simulink model "proto1"  (R2013b)
settings: Solver=ode45  StartTime=0.0  StopTime=20  RelTol=1e-3
libraries: xbsIndex_r4 x145, xps_library x1
settings Model: Creator=root  LastModifiedBy=root

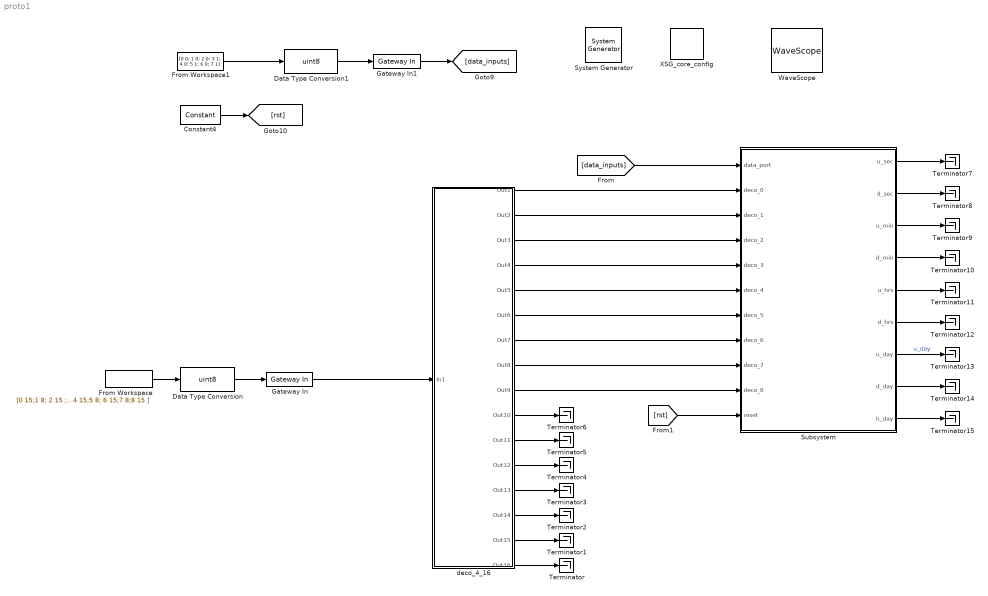
== system proto1 ==
  " System Generator" : xbsIndex_r4/ System Generator  Tag=genX  xilinxfamily=Kintex7  part=xc7k325t  speed=-3  package=fbg676  synthesis_tool=XST  clock_wrapper=Clock Enables  directory=./netlist  proj_type=Project Navigator  Synth_file=XST Defaults  Impl_file=ISE Defaults  testbench=off  simulink_period=1  sysclk_period=10  dcm_input_clock_period=10  incr_netlist=off  trim_vbits=Everywhere in SubSystem  dbl_ovrd=According to Block Masks  core_generation=According to Block Masks  run_coregen=off  deprecated_control=off  eval_field=0  block_type=sysgen
  Constant4 : xbsIndex_r4/Constant  const=0  gui_display_data_type=Boolean  arith_type=Boolean  n_bits=16  bin_pt=14  preci_type=Single  exp_width=8  frac_width=24  explicit_period=on  period=1  equ=P=C  opselect=C  inp2=PCIN>>17  opr=+  inp1=P  carry=CIN  dbl_ovrd=off  block_type=constant
  Data Type Conversion : DataTypeConversion  OutDataTypeStr=uint8
  Data Type Conversion1 : DataTypeConversion  OutDataTypeStr=uint8
  From Workspace : FromWorkspace  VariableName=[0 15;1 8; 2 15 ;3 8; 4 15;5 8; 6 15;7 8;8 15 ]  OutDataTypeStr=double  SampleTime=0  OutputAfterFinalValue=Holding final value
  From Workspace1 : FromWorkspace  VariableName=[0 0; 1 0; 2 0; 3 1; 4 0; 5 1; 6 0; 7 1]  OutDataTypeStr=double  SampleTime=0  OutputAfterFinalValue=Holding final value
  Gateway In : xbsIndex_r4/Gateway In  gui_display_data_type=Fixed-point  arith_type=Unsigned  n_bits=8  bin_pt=0  preci_type=Single  exp_width=8  frac_width=24  quantization="Round  (unbiased: +/- Inf)"  overflow=Saturate  period=1  dbl_ovrd=off  timing_constraint=None  locs_specified=off  LOCs={}  UseAsADC=off  ADCChannel='1'  inherit_from_input=off  hdl_port=on  block_type=gatewayin
  Gateway In1 : xbsIndex_r4/Gateway In  gui_display_data_type=Fixed-point  arith_type=Unsigned  n_bits=8  bin_pt=0  preci_type=Single  exp_width=8  frac_width=24  quantization="Round  (unbiased: +/- Inf)"  overflow=Saturate  period=1  dbl_ovrd=off  timing_constraint=None  locs_specified=off  LOCs={}  UseAsADC=off  ADCChannel='1'  inherit_from_input=off  hdl_port=on  block_type=gatewayin
  Subsystem : Subsystem
  Terminator{,1..15} (16 alike) : Terminator
  WaveScope : xbsIndex_r4/WaveScope  block_type=wavescope
  XSG_core_config : xps_library/XSG_core_config  Tag=xps:xsg  hw_sys=ROACH2:sx475t  clk_src=sys_clk  ROACH_clk_src=sys_clk  ROACH2_clk_src=sys_clk  MKDIG_clk_src=sys_clk  clk_rate=100  sample_period=1  synthesis_tool=XST
  deco_4_16 : Subsystem
  wires:
  From Workspace/1 -> Data Type Conversion/1
  Data Type Conversion/1 -> Gateway In/1
  Gateway In/1 -> deco_4_16/1(In1)
  deco_4_16/16(Out16) -> Terminator/1
  deco_4_16/15(Out15) -> Terminator1/1
  deco_4_16/14(Out14) -> Terminator2/1
  deco_4_16/13(Out13) -> Terminator3/1
  deco_4_16/12(Out12) -> Terminator4/1
  deco_4_16/11(Out11) -> Terminator5/1
  deco_4_16/10(Out10) -> Terminator6/1
  deco_4_16/1(Out1) -> Subsystem/2(deco_0)
  deco_4_16/2(Out2) -> Subsystem/3(deco_1)
  deco_4_16/3(Out3) -> Subsystem/4(deco_2)
  deco_4_16/4(Out4) -> Subsystem/5(deco_3)
  deco_4_16/5(Out5) -> Subsystem/6(deco_4)
  deco_4_16/6(Out6) -> Subsystem/7(deco_5)
  deco_4_16/7(Out7) -> Subsystem/8(deco_6)
  deco_4_16/8(Out8) -> Subsystem/9(deco_7)
  deco_4_16/9(Out9) -> Subsystem/10(deco_8)
  From Workspace1/1 -> Data Type Conversion1/1
  Data Type Conversion1/1 -> Gateway In1/1
  Gateway In1/1 -> [data_inputs]
  Constant4/1 -> [rst]
  [data_inputs] -> Subsystem/1(data_port)
  [rst] -> Subsystem/11(reset)
  Subsystem/1(u_sec) -> Terminator7/1
  Subsystem/2(d_sec) -> Terminator8/1
  Subsystem/3(u_min) -> Terminator9/1
  Subsystem/4(d_min) -> Terminator10/1
  Subsystem/5(u_hrs) -> Terminator11/1
  Subsystem/6(d_hrs) -> Terminator12/1
  Subsystem/7(u_day) -> Terminator13/1  "u_day"
  Subsystem/8(d_day) -> Terminator14/1
  Subsystem/9(h_day) -> Terminator15/1

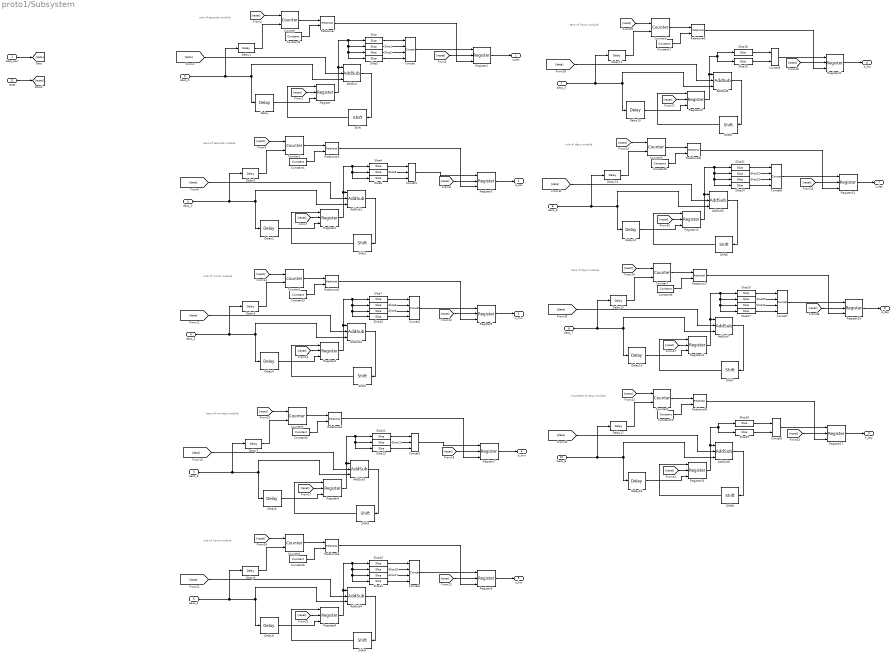
== system proto1/Subsystem ==
  note: unit of seconds module
  note: tens of seconds module
  note: unit of minits module
  note: tens of minutes module
  note: unit of hours module
  note: tens of hours module
  note: unit of days module
  note: tens of days module
  note: houdreds of days module
  data_port : Inport
  deco_0 : Inport  Port=2
  deco_1 : Inport  Port=3
  deco_2 : Inport  Port=4
  deco_3 : Inport  Port=5
  deco_4 : Inport  Port=6
  deco_5 : Inport  Port=7
  deco_6 : Inport  Port=8
  deco_7 : Inport  Port=9
  deco_8 : Inport  Port=10
  reset : Inport  Port=11
  AddSub{,2,4,6..7} (5 alike) : xbsIndex_r4/AddSub  mode=Addition  use_carryin=off  use_carryout=off  en=on  latency=1  precision=User Defined  arith_type=Unsigned  n_bits=5  bin_pt=0  quantization=Truncate  overflow=Wrap  dbl_ovrd=off  use_behavioral_HDL=off  hw_selection=Fabric  pipelined=off  block_type=addsub
  AddSub1 : xbsIndex_r4/AddSub  mode=Addition  use_carryin=off  use_carryout=off  en=on  latency=1  precision=User Defined  arith_type=Unsigned  n_bits=4  bin_pt=0  quantization=Truncate  overflow=Wrap  dbl_ovrd=off  use_behavioral_HDL=off  hw_selection=Fabric  pipelined=off  block_type=addsub
  AddSub3 : xbsIndex_r4/AddSub  mode=Addition  use_carryin=off  use_carryout=off  en=on  latency=1  precision=User Defined  arith_type=Unsigned  n_bits=4  bin_pt=0  quantization=Truncate  overflow=Wrap  dbl_ovrd=off  use_behavioral_HDL=off  hw_selection=Fabric  pipelined=off  block_type=addsub
  AddSub5 : xbsIndex_r4/AddSub  mode=Addition  use_carryin=off  use_carryout=off  en=on  latency=1  precision=User Defined  arith_type=Unsigned  n_bits=3  bin_pt=0  quantization=Truncate  overflow=Wrap  dbl_ovrd=off  use_behavioral_HDL=off  hw_selection=Fabric  pipelined=off  block_type=addsub
  AddSub8 : xbsIndex_r4/AddSub  mode=Addition  use_carryin=off  use_carryout=off  en=on  latency=1  precision=User Defined  arith_type=Unsigned  n_bits=3  bin_pt=0  quantization=Truncate  overflow=Wrap  dbl_ovrd=off  use_behavioral_HDL=off  hw_selection=Fabric  pipelined=off  block_type=addsub
  Concat{,2,4,6..7} (5 alike) : xbsIndex_r4/Concat  num_inputs=4  dbl_ovrd=off  block_type=concat
  Concat1 : xbsIndex_r4/Concat  num_inputs=3  dbl_ovrd=off  block_type=concat
  Concat3 : xbsIndex_r4/Concat  num_inputs=3  dbl_ovrd=off  block_type=concat
  Concat5 : xbsIndex_r4/Concat  num_inputs=2  dbl_ovrd=off  block_type=concat
  Concat8 : xbsIndex_r4/Concat  num_inputs=2  dbl_ovrd=off  block_type=concat
  Constant1 : xbsIndex_r4/Constant  const=3  gui_display_data_type=Fixed-point  arith_type=Unsigned  n_bits=4  bin_pt=0  preci_type=Single  exp_width=8  frac_width=24  explicit_period=on  period=1  equ=P=C  opselect=C  inp2=PCIN>>17  opr=+  inp1=P  carry=CIN  dbl_ovrd=off  block_type=constant
  Constant10 : xbsIndex_r4/Constant  const=2  gui_display_data_type=Fixed-point  arith_type=Unsigned  n_bits=3  bin_pt=0  preci_type=Single  exp_width=8  frac_width=24  explicit_period=on  period=1  equ=P=C  opselect=C  inp2=PCIN>>17  opr=+  inp1=P  carry=CIN  dbl_ovrd=off  block_type=constant
  Constant{2..3,6,8..9} (5 alike) : xbsIndex_r4/Constant  const=4  gui_display_data_type=Fixed-point  arith_type=Unsigned  n_bits=4  bin_pt=0  preci_type=Single  exp_width=8  frac_width=24  explicit_period=on  period=1  equ=P=C  opselect=C  inp2=PCIN>>17  opr=+  inp1=P  carry=CIN  dbl_ovrd=off  block_type=constant
  Constant5 : xbsIndex_r4/Constant  const=3  gui_display_data_type=Fixed-point  arith_type=Unsigned  n_bits=4  bin_pt=0  preci_type=Single  exp_width=8  frac_width=24  explicit_period=on  period=1  equ=P=C  opselect=C  inp2=PCIN>>17  opr=+  inp1=P  carry=CIN  dbl_ovrd=off  block_type=constant
  Constant7 : xbsIndex_r4/Constant  const=2  gui_display_data_type=Fixed-point  arith_type=Unsigned  n_bits=3  bin_pt=0  preci_type=Single  exp_width=8  frac_width=24  explicit_period=on  period=1  equ=P=C  opselect=C  inp2=PCIN>>17  opr=+  inp1=P  carry=CIN  dbl_ovrd=off  block_type=constant
  Counter{,1..8} (9 alike) : xbsIndex_r4/Counter  cnt_type=Free Running  cnt_to=Inf  operation=Up  start_count=0  cnt_by_val=1  arith_type=Unsigned  n_bits=4  bin_pt=0  load_pin=off  rst=on  en=on  explicit_period=on  period=1  dbl_ovrd=off  use_behavioral_HDL=off  implementation=Fabric  block_type=counter
  Delay{,1..17} (18 alike) : xbsIndex_r4/Delay  rst=off  infoeditControl=Selection of Reset will increase slice count due to use of real FFs and instead of SRLs  en=off  latency=1  dbl_ovrd=off  reg_retiming=off  block_type=delay
  Register{,1..17} (18 alike) : xbsIndex_r4/Register  init=0  rst=on  en=on  dbl_ovrd=off  block_type=register
  Relational{,1..8} (9 alike) : xbsIndex_r4/Relational  mode=a=b  en=off  latency=0  dbl_ovrd=off  block_type=relational
  Shift{,1..8} (9 alike) : xbsIndex_r4/Shift  shift_dir=Left  shift_bits=1  en=off  latency=0  precision=Full  arith_type="Signed  (2's comp)"  n_bits=16  bin_pt=14  quantization=Truncate  overflow=Wrap  dbl_ovrd=off  block_type=shift
  Slice{,4,7,11,15,18,20..21,28} (9 alike) : xbsIndex_r4/Slice  nbits=1  boolean_output=off  mode=Lower Bit Location + Width  bit1=0  base1=MSB of Input  bit0=1  base0=LSB of Input  dbl_ovrd=off  block_type=slice
  Slice{1,5,8,12,16,19,22,25,29} (9 alike) : xbsIndex_r4/Slice  nbits=1  boolean_output=off  mode=Lower Bit Location + Width  bit1=0  base1=MSB of Input  bit0=2  base0=LSB of Input  dbl_ovrd=off  block_type=slice
  Slice{3,10,14,24,27} (5 alike) : xbsIndex_r4/Slice  nbits=1  boolean_output=off  mode=Lower Bit Location + Width  bit1=0  base1=MSB of Input  bit0=4  base0=LSB of Input  dbl_ovrd=off  block_type=slice
  Slice{2,6,9,13,17,23,26} (7 alike) : xbsIndex_r4/Slice  nbits=1  boolean_output=off  mode=Lower Bit Location + Width  bit1=0  base1=MSB of Input  bit0=3  base0=LSB of Input  dbl_ovrd=off  block_type=slice
  u_sec : Outport
  d_sec : Outport  Port=2
  u_min : Outport  Port=3
  d_min : Outport  Port=4
  u_hrs : Outport  Port=5
  d_hrs : Outport  Port=6
  u_day : Outport  Port=7
  d_day : Outport  Port=8
  h_day : Outport  Port=9
  wires:
  Constant7/1 -> Relational5/2
  Shift7/1 -> Register14/1
  Delay14/1 -> Register14/3
  [reset] -> Register10/2
  deco_5/1 -> Delay11/1, Delay10/1, AddSub5/3
  Register12/1 -> Slice24/1, Slice23/1, Slice22/1, Slice21/1, AddSub6/1
  Shift5/1 -> Register10/1
  Relational5/1 -> Register11/3
  [reset] -> Counter5/1
  Register15/1 -> d_day/1
  Delay15/1 -> Counter7/2
  [data] -> AddSub1/2
  Register13/1 -> u_day/1
  Delay13/1 -> Counter6/2
  Slice24/1 -> Concat6/4
  Register11/1 -> d_hrs/1
  [data] -> AddSub5/2
  AddSub5/1 -> Shift5/1
  Slice21/1 -> Concat6/1
  Slice23/1 -> Concat6/3
  Slice22/1 -> Concat6/2
  Register5/1 -> u_min/1
  Shift2/1 -> Register4/1
  [reset] -> Register3/2
  Slice7/1 -> Concat2/1
  Slice8/1 -> Concat2/2
  Delay6/1 -> Register6/3
  Slice12/1 -> Concat3/2
  [data] -> AddSub7/2
  [reset] -> Register11/2
  Register3/1 -> d_sec/1
  Counter7/1 -> Relational7/1
  Delay/1 -> Register/3
  Slice/1 -> Concat/1
  Slice1/1 -> Concat/2
  Slice2/1 -> Concat/3
  Concat/1 -> Register1/1
  [reset] -> Counter/1
  Counter/1 -> Relational/1
  Constant2/1 -> Relational/2
  Relational/1 -> Register1/3
  [reset] -> Register1/2
  Register1/1 -> u_sec/1
  Delay1/1 -> Counter/2
  Slice6/1 -> Concat1/3
  [reset] -> Counter2/1
  Slice27/1 -> Concat7/4
  Slice20/1 -> Concat7/1
  Slice25/1 -> Concat7/2
  Slice26/1 -> Concat7/3
  Relational8/1 -> Register17/3
  [reset] -> Register17/2
  Register17/1 -> h_day/1
  Delay17/1 -> Counter8/2
  Register8/1 -> Slice14/1, Slice17/1, Slice16/1, Slice15/1, AddSub4/1
  [reset] -> Register12/2
  Shift6/1 -> Register12/1
  Delay12/1 -> Register12/3
  Delay10/1 -> Register10/3
  Slice29/1 -> Concat8/2
  Concat8/1 -> Register17/1
  [reset] -> Counter8/1
  Counter8/1 -> Relational8/1
  Constant10/1 -> Relational8/2
  AddSub8/1 -> Shift8/1
  Shift8/1 -> Register16/1
  Delay16/1 -> Register16/3
  Slice28/1 -> Concat8/1
  [reset] -> Register15/2
  deco_8/1 -> Delay17/1, AddSub8/3, Delay16/1
  [data] -> AddSub8/2
  [reset] -> Register16/2
  Register14/1 -> Slice27/1, Slice26/1, Slice25/1, Slice20/1, AddSub7/1
  Constant9/1 -> Relational7/2
  Relational7/1 -> Register15/3
  AddSub7/1 -> Shift7/1
  [reset] -> Register14/2
  Register16/1 -> Slice29/1, Slice28/1, AddSub8/1
  Register2/1 -> Slice6/1, Slice5/1, Slice4/1, AddSub1/1
  Constant5/1 -> Relational3/2
  [reset] -> Register7/2
  Slice19/1 -> Concat5/2
  [reset] -> Register2/2
  Constant1/1 -> Relational1/2
  AddSub2/1 -> Shift2/1
  [reset] -> Register4/2
  Concat7/1 -> Register15/1
  [reset] -> Counter7/1
  deco_2/1 -> Delay5/1, Delay4/1, AddSub2/3
  [data] -> AddSub3/2
  Delay4/1 -> Register4/3
  Slice9/1 -> Concat2/3
  Counter1/1 -> Relational1/1
  Counter5/1 -> Relational5/1
  Concat1/1 -> Register3/1
  Slice3/1 -> Concat/4
  Shift3/1 -> Register6/1
  AddSub3/1 -> Shift3/1
  Register10/1 -> Slice19/1, Slice18/1, AddSub5/1
  Relational2/1 -> Register5/3
  [reset] -> Register5/2
  AddSub1/1 -> Shift1/1
  Delay7/1 -> Counter3/2
  [data] -> AddSub6/2
  AddSub6/1 -> Shift6/1
  Relational3/1 -> Register7/3
  Register7/1 -> d_min/1
  deco_3/1 -> Delay7/1, Delay6/1, AddSub3/3
  Counter3/1 -> Relational3/1
  [reset] -> Counter3/1
  Slice10/1 -> Concat2/4
  Delay5/1 -> Counter2/2
  [data] -> AddSub2/2
  Relational1/1 -> Register3/3
  Counter2/1 -> Relational2/1
  Constant3/1 -> Relational2/2
  [reset] -> Register9/2
  Register9/1 -> u_hrs/1
  Delay9/1 -> Counter4/2
  Slice14/1 -> Concat4/4
  Register/1 -> Slice3/1, Slice2/1, Slice1/1, Slice/1, AddSub/1
  Register6/1 -> Slice13/1, Slice12/1, Slice11/1, AddSub3/1
  Concat2/1 -> Register5/1
  Delay3/1 -> Counter1/2
  Register4/1 -> Slice10/1, Slice9/1, Slice8/1, Slice7/1, AddSub2/1
  [reset] -> Counter4/1
  deco_6/1 -> Delay13/1, AddSub6/3, Delay12/1
  [data] -> AddSub4/2
  AddSub4/1 -> Shift4/1
  [reset] -> Register8/2
  deco_4/1 -> Delay9/1, Delay8/1, AddSub4/3
  Concat5/1 -> Register11/1
  Constant8/1 -> Relational6/2
  [reset] -> Register13/2
  Relational6/1 -> Register13/3
  Slice17/1 -> Concat4/3
  Constant6/1 -> Relational4/2
  Counter4/1 -> Relational4/1
  Relational4/1 -> Register9/3
  Delay11/1 -> Counter5/2
  Concat6/1 -> Register13/1
  Counter6/1 -> Relational6/1
  [reset] -> Counter6/1
  Slice18/1 -> Concat5/1
  deco_7/1 -> Delay15/1, Delay14/1, AddSub7/3
  Shift4/1 -> Register8/1
  Delay8/1 -> Register8/3
  Slice15/1 -> Concat4/1
  Concat4/1 -> Register9/1
  Slice16/1 -> Concat4/2
  Slice13/1 -> Concat3/3
  Concat3/1 -> Register7/1
  deco_1/1 -> Delay3/1, Delay2/1, AddSub1/3
  Delay2/1 -> Register2/3
  deco_0/1 -> Delay1/1, Delay/1, AddSub/3
  [data] -> AddSub/2
  AddSub/1 -> Shift/1
  [reset] -> Register/2
  Shift/1 -> Register/1
  Slice5/1 -> Concat1/2
  Shift1/1 -> Register2/1
  Slice4/1 -> Concat1/1
  [reset] -> Register6/2
  Slice11/1 -> Concat3/1
  [reset] -> Counter1/1
  data_port/1 -> [data]
  reset/1 -> [reset]

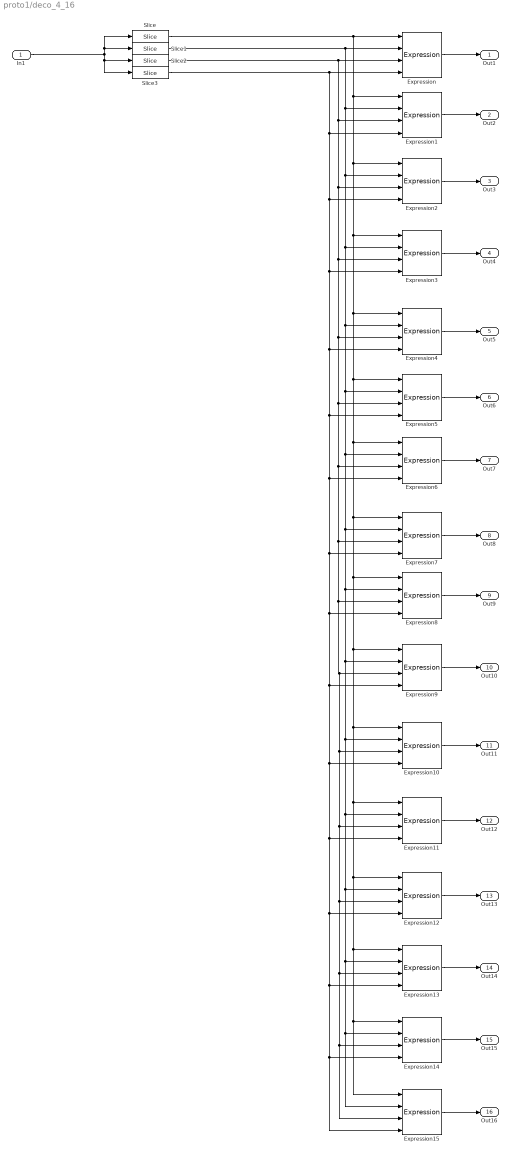
== system proto1/deco_4_16 ==
  In1 : Inport
  Expression : xbsIndex_r4/Expression  expression=~a & ~b & ~c & ~d  align_bp=on  en=off  latency=0  precision=Full  arith_type=Unsigned  n_bits=16  bin_pt=0  dbl_ovrd=off  block_type=expr
  Expression1 : xbsIndex_r4/Expression  expression=~a & ~b & ~c & d  align_bp=on  en=off  latency=0  precision=Full  arith_type=Unsigned  n_bits=16  bin_pt=0  dbl_ovrd=off  block_type=expr
  Expression10 : xbsIndex_r4/Expression  expression=a & ~b & c & ~d  align_bp=on  en=off  latency=0  precision=Full  arith_type=Unsigned  n_bits=16  bin_pt=0  dbl_ovrd=off  block_type=expr
  Expression11 : xbsIndex_r4/Expression  expression=a & ~b & c & d  align_bp=on  en=off  latency=0  precision=Full  arith_type=Unsigned  n_bits=16  bin_pt=0  dbl_ovrd=off  block_type=expr
  Expression12 : xbsIndex_r4/Expression  expression=a & b & ~c & ~d  align_bp=off  en=off  latency=0  precision=Full  arith_type=Unsigned  n_bits=16  bin_pt=0  dbl_ovrd=off  block_type=expr
  Expression13 : xbsIndex_r4/Expression  expression=a & b & ~c & d  align_bp=off  en=off  latency=0  precision=Full  arith_type=Unsigned  n_bits=16  bin_pt=0  dbl_ovrd=off  block_type=expr
  Expression14 : xbsIndex_r4/Expression  expression=a & b & c & ~d  align_bp=off  en=off  latency=0  precision=Full  arith_type=Unsigned  n_bits=16  bin_pt=0  dbl_ovrd=off  block_type=expr
  Expression15 : xbsIndex_r4/Expression  expression=a & b & c & d  align_bp=off  en=off  latency=0  precision=Full  arith_type=Unsigned  n_bits=16  bin_pt=0  dbl_ovrd=off  block_type=expr
  Expression2 : xbsIndex_r4/Expression  expression=~a & ~b & c & ~d  align_bp=on  en=off  latency=0  precision=Full  arith_type=Unsigned  n_bits=16  bin_pt=0  dbl_ovrd=off  block_type=expr
  Expression3 : xbsIndex_r4/Expression  expression=~a & ~b & c & d  align_bp=on  en=off  latency=0  precision=Full  arith_type=Unsigned  n_bits=16  bin_pt=0  dbl_ovrd=off  block_type=expr
  Expression4 : xbsIndex_r4/Expression  expression=~a & b & ~c & ~d  align_bp=on  en=off  latency=0  precision=Full  arith_type=Unsigned  n_bits=16  bin_pt=0  dbl_ovrd=off  block_type=expr
  Expression5 : xbsIndex_r4/Expression  expression=~a & b & ~c & d  align_bp=on  en=off  latency=0  precision=Full  arith_type=Unsigned  n_bits=16  bin_pt=0  dbl_ovrd=off  block_type=expr
  Expression6 : xbsIndex_r4/Expression  expression=~a & b & c & ~d  align_bp=on  en=off  latency=0  precision=Full  arith_type=Unsigned  n_bits=16  bin_pt=0  dbl_ovrd=off  block_type=expr
  Expression7 : xbsIndex_r4/Expression  expression=~a & b & c & d  align_bp=on  en=off  latency=0  precision=Full  arith_type=Unsigned  n_bits=16  bin_pt=0  dbl_ovrd=off  block_type=expr
  Expression8 : xbsIndex_r4/Expression  expression=a & ~b & ~c & ~d  align_bp=on  en=off  latency=0  precision=Full  arith_type=Unsigned  n_bits=16  bin_pt=0  dbl_ovrd=off  block_type=expr
  Expression9 : xbsIndex_r4/Expression  expression=a & ~b & ~c & d  align_bp=on  en=off  latency=0  precision=Full  arith_type=Unsigned  n_bits=16  bin_pt=0  dbl_ovrd=off  block_type=expr
  Slice : xbsIndex_r4/Slice  nbits=1  boolean_output=on  mode=Lower Bit Location + Width  bit1=0  base1=MSB of Input  bit0=3  base0=LSB of Input  dbl_ovrd=off  block_type=slice
  Slice1 : xbsIndex_r4/Slice  nbits=1  boolean_output=on  mode=Lower Bit Location + Width  bit1=2  base1=LSB of Input  bit0=2  base0=LSB of Input  dbl_ovrd=off  block_type=slice
  Slice2 : xbsIndex_r4/Slice  nbits=1  boolean_output=on  mode=Lower Bit Location + Width  bit1=1  base1=LSB of Input  bit0=1  base0=LSB of Input  dbl_ovrd=off  block_type=slice
  Slice3 : xbsIndex_r4/Slice  nbits=1  boolean_output=on  mode=Lower Bit Location + Width  bit1=0  base1=LSB of Input  bit0=0  base0=LSB of Input  dbl_ovrd=off  block_type=slice
  Out1 : Outport
  Out2 : Outport  Port=2
  Out3 : Outport  Port=3
  Out4 : Outport  Port=4
  Out5 : Outport  Port=5
  Out6 : Outport  Port=6
  Out7 : Outport  Port=7
  Out8 : Outport  Port=8
  Out9 : Outport  Port=9
  Out10 : Outport  Port=10
  Out11 : Outport  Port=11
  Out12 : Outport  Port=12
  Out13 : Outport  Port=13
  Out14 : Outport  Port=14
  Out15 : Outport  Port=15
  Out16 : Outport  Port=16
  wires:
  Expression13/1 -> Out14/1
  Expression14/1 -> Out15/1
  Expression15/1 -> Out16/1
  Slice2/1 -> Expression2/3, Expression3/3, Expression4/3, Expression5/3, Expression6/3, Expression7/3, Expression8/3, Expression10/3, Expression11/3, Expression12/3, Expression13/3, Expression14/3, Expression15/3, Expression9/3, Expression1/3, Expression/3
  Expression10/1 -> Out11/1
  Slice3/1 -> Expression1/4, Expression2/4, Expression3/4, Expression4/4, Expression5/4, Expression6/4, Expression7/4, Expression8/4, Expression11/4, Expression13/4, Expression14/4, Expression15/4, Expression12/4, Expression10/4, Expression9/4, Expression/4
  Expression11/1 -> Out12/1
  Expression12/1 -> Out13/1
  In1/1 -> Slice3/1, Slice2/1, Slice/1, Slice1/1
  Expression/1 -> Out1/1
  Expression1/1 -> Out2/1
  Expression2/1 -> Out3/1
  Expression3/1 -> Out4/1
  Expression4/1 -> Out5/1
  Expression5/1 -> Out6/1
  Expression6/1 -> Out7/1
  Expression7/1 -> Out8/1
  Expression8/1 -> Out9/1
  Expression9/1 -> Out10/1
  Slice/1 -> Expression3/1, Expression4/1, Expression5/1, Expression6/1, Expression7/1, Expression10/1, Expression11/1, Expression13/1, Expression14/1, Expression15/1, Expression12/1, Expression9/1, Expression8/1, Expression2/1, Expression1/1, Expression/1
  Slice1/1 -> Expression1/2, Expression2/2, Expression3/2, Expression4/2, Expression5/2, Expression6/2, Expression7/2, Expression8/2, Expression10/2, Expression11/2, Expression12/2, Expression13/2, Expression14/2, Expression15/2, Expression9/2, Expression/2
